simulink model "Modelo_lineal_5GDL_2022"  (R2021b)
settings: Solver=VariableStepAuto  StartTime=0.0  StopTime=0.1  MaxStep=1e-5  RelTol=1e-6
values from neighbouring files (symbols this model uses):
  g = 9.81    [main.m]
undefined symbols (not defined in the file or in its folder): A_EMS, A_HEMS, AG0, B_EMS, B_HEMS, beta, C_EMS, C_HEMS, D_EMS, D_HEMS, dTSensor, filterConstant, I_front, I_rear, initial_conds, noiseSensor, pod, ROTX_0, ROTY_0, ROTZ_0, y_ini, z_0, z_ini
libraries: shared6dof x1
(part 2 of 2)

== matlab function Modelo_lineal_5GDL_2022/Non-linear 6 DOF model/MATLAB Function2 ==
  data: airgaps input; u_1 input; u output; pod parameter; beta parameter
function u  = ag2pos(airgaps, u_1, pod, beta)
% Computes the position and attitute od the pod as a function of the airgaps 
% ═════════════════════════════════════════════════════════════════════════
% Last updated: 27.01.2022
% ═════════════════════════════════════════════════════════════════════════
% INPUT:
%   airgaps   = Vector with airgaps in [m]. The 6 first values correspond
%               to the levitation units, and the 4 last values correspond 
%               to guidance. 
%               Size 10 x 1
%   beta      = Measure acceptance tolerance [-]
%               Scalar
%   pod       = Struct containing data about
%                   *mass (Mass and inertia)
%                   *brakes (Pressures, friction coefficients and forces)
%                   *levitation (Maps of forces)
%                   *guiding (Maps of forces)
%                   *propulsion (Force as a function of velocity). 
%                   *geometry (points of application of forces wrt CG)
%                   *general (simulation parameters)
%   u         = DOF vector in (t-1), containing the estimations of the 
%               position in the y and z directions [m] and the 3 rotation 
%               angles [rad]
%               Size 5 x 1
% OUTPUT:
%   u         = DOF vector, containing the estimations of the position in
%               the y and z directions [m] and the 3 rotation angles [rad]
%               Size 5 x 1
% ═════════════════════════════════════════════════════════════════════════


%%% Input check (4 inputs)
narginchk(4,4);

%%% Ensure inputs are well defined
% airgaps must be a 10 dimensional vector
if ~ismatrix(airgaps) || numel(airgaps) ~= 10
    error('Vector with airgaps is not properly defined');
end

% % Filter incorrect measures
% if any(isnan(airgaps))
%     warning('Signal of unit number %d is incorrect. The system will ignore it, but computation will be slower.', find(isnan(airgaps)));
%     airgaps(isnan(airgaps)) = 0;
% end

% % Beta must be scalar
% if ~(isscalar(beta))
%     error('beta must be an scalar')
% end


%%% Auxiliar vectors initialization 
coder.varsize('y_aux'); 
coder.varsize('z_aux'); 
coder.varsize('rotx_aux');
coder.varsize('roty_aux');
coder.varsize('rotz_aux')
coder.varsize('malfunction'); 

y_aux       = zeros(4,1);
idx_y       = false(4,1);
z_aux       = zeros(6,1);
idx_z       = false(6,1);
rotx_aux    = zeros(3,1);
idxx        = false(3,1);
roty_aux    = zeros(6,1);
idxy        = false(6,1);
rotz_aux    = zeros(2,1);
idxz        = false(2,1);
malfunction = true(11,1);
y = 0; z = 0; rotx = 0; roty = 0; rotz = 0;

%%% Attitude
rotx_aux(1) = asin((airgaps(1) - airgaps(4))/(2 * pod.geometry.y_LEV));
rotx_aux(2) = asin((airgaps(2) - airgaps(5))/(2 * pod.geometry.y_LEV));
rotx_aux(3) = asin((airgaps(3) - airgaps(6))/(2 * pod.geometry.y_LEV));

roty_aux(1) = asin((airgaps(5) - airgaps(4))/(    pod.geometry.z_LEV));
roty_aux(2) = asin((airgaps(6) - airgaps(4))/(2 * pod.geometry.z_LEV));
roty_aux(3) = asin((airgaps(6) - airgaps(5))/(    pod.geometry.z_LEV));
roty_aux(4) = asin((airgaps(3) - airgaps(2))/(    pod.geometry.z_LEV));
roty_aux(5) = asin((airgaps(3) - airgaps(1))/(2 * pod.geometry.z_LEV));
roty_aux(6) = asin((airgaps(2) - airgaps(1))/(    pod.geometry.z_LEV));

rotz_aux(1) = asin((airgaps(8) - airgaps(7 ))/(pod.geometry.x_G_front + pod.geometry.x_G_rear));
rotz_aux(1) = asin((airgaps(9) - airgaps(10))/(pod.geometry.x_G_front + pod.geometry.x_G_rear));

while any(malfunction)
    rotx = mean(rotx_aux);
    roty = mean(roty_aux);
    rotz = mean(rotz_aux);

    resx = abs(rotx_aux - rotx);
    resy = abs(roty_aux - roty);
    resz = abs(rotz_aux - rotz);

    idxx =  (resx> abs(beta*rotx));
    idxy =  (resy> abs(beta*roty));
    idxz =  (resz> abs(beta*rotz));

    malfunction = [idxx; idxy; idxz];

    rotx_aux = rotx_aux(~(idxx));
    roty_aux = roty_aux(~(idxy));
    rotz_aux = rotz_aux(~(idxz));
end

malfunction = true(10,1);

%%% Position
x_G     = 0.5 * (pod.geometry.x_G_front + pod.geometry.x_G_rear);
x_LEV   = 0.5 * (pod.geometry.x_LEV_front + pod.geometry.x_LEV_rear);

y_aux(1) = airgaps(7)    + pod.geometry.y_G * cos(rotz) +   x_G * sin(rotz);
y_aux(2) = airgaps(8)    + pod.geometry.y_G * cos(rotz) -   x_G * sin(rotz);
y_aux(3) = - airgaps(9)  - pod.geometry.y_G * cos(rotz) - x_G * sin(rotz);
y_aux(4) = - airgaps(10) - pod.geometry.y_G * cos(rotz) + x_G * sin(rotz);

z_aux(1) = airgaps(1)  + pod.geometry.z_LEV * cos(roty) + x_LEV * sin(roty) - pod.geometry.y_LEV * sin(rotx);
z_aux(2) = airgaps(2)  + pod.geometry.z_LEV * cos(roty)                     - pod.geometry.y_LEV * sin(rotx);
z_aux(3) = airgaps(3)  + pod.geometry.z_LEV * cos(roty) - x_LEV * sin(roty) - pod.geometry.y_LEV * sin(rotx);
z_aux(4) = airgaps(4)  + pod.geometry.z_LEV * cos(roty) + x_LEV * sin(roty) + pod.geometry.y_LEV * sin(rotx);
z_aux(5) = airgaps(5)  + pod.geometry.z_LEV * cos(roty)                     + pod.geometry.y_LEV * sin(rotx);
z_aux(6) = airgaps(6)  + pod.geometry.z_LEV * cos(roty) - x_LEV * sin(roty) + pod.geometry.y_LEV * sin(rotx);


while any(malfunction)
    y = mean(y_aux);
    z = mean(z_aux);

    resy = abs(y_aux - y);
    resz = abs(z_aux - z);

    idx_y = (resy>beta*y);
    idx_z = (resz>beta*z);

    malfunction = [idxy; idxz];

    y_aux = y_aux(~(idx_y));
    z_aux = z_aux(~(idx_z));
end

u = [y, z, rotx, roty, rotz]';

u(isnan(u)) = u_1(isnan(u));

end

== matlab function Modelo_lineal_5GDL_2022/MODELO NOLINEAL SIMPLIFICADO/Modelo_5DOF/MATLAB Function1 ==
  data: airgap input; F output; intensity input; pod parameter
function F = HEMSlev(airgap, intensity, pod)
% Computes the levitation force (N) of all the HEMS units as a function of 
% their air gaps (mm) and intensities (A)
% ═════════════════════════════════════════════════════════════════════════
% Last updated: 15.12.2021
% ════════════════════════════════════════════════════════════════════════

x   = airgap(1:6);
y   = intensity(1:6);

F = pod.levitation.poly_1_unit.p00 + ...
    pod.levitation.poly_1_unit.p10.*x + ...
    pod.levitation.poly_1_unit.p01.*y + ...
    pod.levitation.poly_1_unit.p20.*x.^2 + ...
    pod.levitation.poly_1_unit.p11.*x.*y + ...
    pod.levitation.poly_1_unit.p02.*y.^2 + ...
    pod.levitation.poly_1_unit.p21.*x.^2.*y + ...
    pod.levitation.poly_1_unit.p12.*x.*y.^2 + ...
    pod.levitation.poly_1_unit.p03.*y.^3;

== matlab function Modelo_lineal_5GDL_2022/MODELO NOLINEAL SIMPLIFICADO/Modelo_5DOF/MATLAB Function2 ==
  data: airgap input; F output; intensity input; pod parameter
function F = EMSlev(airgap, intensity, pod)
% Computes the levitation force (N) of all the EMS units as a function of 
% their air gaps (mm) and intensities (A)
% ═════════════════════════════════════════════════════════════════════════
% Last updated: 24.03.2022
% ════════════════════════════════════════════════════════════════════════

x   = airgap(7:10);
y   = intensity(7:10);

F = pod.guiding.poly.p00 + ...
    pod.guiding.poly.p10.*x + ...
    pod.guiding.poly.p01.*y + ...
    pod.guiding.poly.p20.*x.^2 + ...
    pod.guiding.poly.p11.*x.*y + ...
    pod.guiding.poly.p02.*y.^2 + ...
    pod.guiding.poly.p21.*x.^2.*y + ...
    pod.guiding.poly.p12.*x.*y.^2 + ...
    pod.guiding.poly.p03.*y.^3 + ...
    pod.guiding.poly.p22.*x.^2.*y.^2 + ...
    pod.guiding.poly.p13.*x.*y.^3 + ...
    pod.guiding.poly.p04.*y.^4 + ...
    pod.guiding.poly.p23.*x.^2.*y.^3 + ...
    pod.guiding.poly.p14.*x.*y.^4 + ...
    pod.guiding.poly.p05.*y.^5;

== matlab function Modelo_lineal_5GDL_2022/Non-linear 6 DOF model/H7 Pod Dynamic model/Levitation/MATLAB Function ==
  data: v input; F output; pod parameter
function F = HEMSdrag(v, pod)
% Computes the drag force (N) of one HEMS unit as a function of the 
% velocity (m/s)
% ═════════════════════════════════════════════════════════════════════════
% Last updated: 15.12.2021
% ═════════════════════════════════════════════════════════════════════════

F = pod.levitation.drag_1_unit.poly.p3*v^3 + ...
    pod.levitation.drag_1_unit.poly.p2*v^2 + ...
    pod.levitation.drag_1_unit.poly.p1*v   ;

== matlab function Modelo_lineal_5GDL_2022/Non-linear 6 DOF model/H7 Pod Dynamic model/Guidance/MATLAB Function ==
  data: v input; F output
function F = EMSdrag(v)
% Computes the drag force (N) of one EMS units as a function of 
% its velocity (m/s)
% ═════════════════════════════════════════════════════════════════════════
% Last updated: 15.12.2021
% ════════════════════════════════════════════════════════════════════════

F = 0;

== matlab function Modelo_lineal_5GDL_2022/Non-linear 6 DOF model/H7 Pod Dynamic model/Guidance/MATLAB Function1 ==
  data: airgap input; F output; intensity input; pod parameter
function F = EMSlev(airgap, intensity, pod)
% Computes the levitation force (N) of all the EMS units as a function of 
% their air gaps (mm) and intensities (A)
% ═════════════════════════════════════════════════════════════════════════
% Last updated: 24.03.2022
% ════════════════════════════════════════════════════════════════════════

x   = airgap(7:10);
y   = intensity(7:10);

F = pod.guiding.poly.p00 + ...
    pod.guiding.poly.p10.*x + ...
    pod.guiding.poly.p01.*y + ...
    pod.guiding.poly.p20.*x.^2 + ...
    pod.guiding.poly.p11.*x.*y + ...
    pod.guiding.poly.p02.*y.^2 + ...
    pod.guiding.poly.p21.*x.^2.*y + ...
    pod.guiding.poly.p12.*x.*y.^2 + ...
    pod.guiding.poly.p03.*y.^3 + ...
    pod.guiding.poly.p22.*x.^2.*y.^2 + ...
    pod.guiding.poly.p13.*x.*y.^3 + ...
    pod.guiding.poly.p04.*y.^4 + ...
    pod.guiding.poly.p23.*x.^2.*y.^3 + ...
    pod.guiding.poly.p14.*x.*y.^4 + ...
    pod.guiding.poly.p05.*y.^5;

== matlab function Modelo_lineal_5GDL_2022/Non-linear 6 DOF model/H7 Pod Dynamic model/LIM/MATLAB Function ==
  data: v input; acceleration_flag input; F output; pod parameter
function F = LIMtraction(v, acceleration_flag, pod)
% Computes the traction force (N) of the LIM as a function of 
% the absolute velocity of the prototype (m/s)
% ═════════════════════════════════════════════════════════════════════════
% Last updated: 20.12.2021
% ═════════════════════════════════════════════════════════════════════════

if acceleration_flag == 1
    F = pod.propulsion.poly.p3*v^3 + ...
        pod.propulsion.poly.p2*v^2 + ...
        pod.propulsion.poly.p1*v   + ...
        pod.propulsion.poly.p0;

else
    F = pod.propulsion.br_poly.p2*v^2 + ...
        pod.propulsion.br_poly.p1*v   + ...
        pod.propulsion.br_poly.p0;
end

== matlab function Modelo_lineal_5GDL_2022/Non-linear 6 DOF model/H7 Pod Dynamic model/LIM/MATLAB Function1 ==
  data: v input; x input; sign output; pod parameter
function sign = LIMdirection(v, x, pod)
% Decides if the LIM force is being applied to accelerate or to brake 
% by comparing the position of the pod with a predefined treshold
% ═════════════════════════════════════════════════════════════════════════
% Last updated: 20.12.2021
% ═════════════════════════════════════════════════════════════════════════

if x >= pod.brakes.d && v > 0    
    sign = -1;
elseif x >= pod.brakes.d && v <= 0
    sign = 0;
else
    sign = 1;
end

== matlab function Modelo_lineal_5GDL_2022/Non-linear 6 DOF model/H7 Pod Dynamic model/Levitation/MATLAB Function1 ==
  data: airgap input; F output; intensity input; pod parameter
function F = HEMSlev(airgap, intensity, pod)
% Computes the levitation force (N) of all the HEMS units as a function of 
% their air gaps (mm) and intensities (A)
% ═════════════════════════════════════════════════════════════════════════
% Last updated: 15.12.2021
% ════════════════════════════════════════════════════════════════════════

x   = airgap(1:6);
y   = intensity(1:6);

F = pod.levitation.poly_1_unit.p00 + ...
    pod.levitation.poly_1_unit.p10.*x + ...
    pod.levitation.poly_1_unit.p01.*y + ...
    pod.levitation.poly_1_unit.p20.*x.^2 + ...
    pod.levitation.poly_1_unit.p11.*x.*y + ...
    pod.levitation.poly_1_unit.p02.*y.^2 + ...
    pod.levitation.poly_1_unit.p21.*x.^2.*y + ...
    pod.levitation.poly_1_unit.p12.*x.*y.^2 + ...
    pod.levitation.poly_1_unit.p03.*y.^3;

== matlab function Modelo_lineal_5GDL_2022/Non-linear 6 DOF model/H7 Pod Dynamic model/MATLAB Function ==
  data: F input; F_e output; attitude input; pod parameter
function F_e = BF2E(F, attitude, pod)
% Computes the total force in absoute axis
% ═════════════════════════════════════════════════════════════════════════
% Last updated: 27.12.2021
% ═════════════════════════════════════════════════════════════════════════
F     = reshape(F, [3 1]);


F_e = attitude * F + pod.mass.mass * [0 0 9.81]';

== matlab function Modelo_lineal_5GDL_2022/Non-linear 6 DOF model/H7 Pod Dynamic model/Wheels/MATLAB Function ==
  data: z input; F output; pod parameter; z_CF output
function [F, z_CF] = rollingFriction(z, pod)
% Computes the rolling resistance force (N) of the wheels. It distinguishes
% 3 cases: 
%   (1) z = 0. Pod touching the ground
%   (2) z = z_max. Pod touching the ceiling. It is assumed no current
%   applied to the HEMS. 
%   (3) Otherwise. Pod levitating. 
% ═════════════════════════════════════════════════════════════════════════
% Last updated: 26.12.2021
% ═════════════════════════════════════════════════════════════════════════

% F_LEV worst case scenario computation
x   = 12; % [mm]
y   = 0;  % [A]

F_LEV = pod.levitation.poly_1_unit.p00 + ...
        pod.levitation.poly_1_unit.p10.*x + ...
        pod.levitation.poly_1_unit.p01.*y + ...
        pod.levitation.poly_1_unit.p20.*x.^2 + ...
        pod.levitation.poly_1_unit.p11.*x.*y + ...
        pod.levitation.poly_1_unit.p02.*y.^2 + ...
        pod.levitation.poly_1_unit.p21.*x.^2.*y + ...
        pod.levitation.poly_1_unit.p12.*x.*y.^2 + ...
        pod.levitation.poly_1_unit.p03.*y.^3;

% Main algorithm
if z == 0
    F_N   = pod.mass.mass * 9.81;
    z_CF  = - pod.geometry.z_CF;
elseif z == pod.general.z_range
    F_N   = 6 * F_LEV - pod.mass.mass * 9.81;
    z_CF  = pod.geometry.z_CF;
else
    F_N   = 0;
    z_CF  = 0;
end

F = pod.wheels.number * pod.wheels.roll_coef * F_N;

== matlab function Modelo_lineal_5GDL_2022/Non-linear 6 DOF model/H7 Pod Dynamic model/Brakes/MATLAB Function ==
  data: x input; velocity input; F output; emergency input; F_N output; pod parameter
function [F, F_N] = brakes_activation(x, velocity, emergency, pod)
% Computes the braking force of the pneumatic actuators if and only if 
%     (1) The emergency flag has been raised
%     (2) The pod is above the acceleration phase distance
% ═════════════════════════════════════════════════════════════════════════
% Last updated: 20.12.2021
% ═════════════════════════════════════════════════════════════════════════

if (emergency == 1 && x >= pod.brakes.d && velocity >= 0)
    F       = pod.brakes.force * ones(pod.brakes.n,1);
    F_N     = pod.brakes.normal_force * ones(pod.brakes.n,1);
else
    F       = zeros(pod.brakes.n,1);
    F_N     = zeros(pod.brakes.n,1);
end
